simulink model "sl_quadrotor"  (R2024b)
settings: Solver=VariableStepAuto  StartTime=0.0  StopTime=7  RelTol=1e-3  EnableMultiTasking=on
PreLoadFcn:
  | % load parameters of the default quadrotor
  | disp('Quadrotor parameters loaded by PreLoadFcn')
  | mdl_quadrotor
undefined symbols (not defined in the file or in its folder): P, quadrotor, rot2
libraries: simulink x3, roblocks x1, robotcorelib x1, uavutilslib x1
settings Model: Creator=corkep  LastModifiedBy=dawid
settings SolverCC: AlgebraicLoopSolver=TrustRegion
settings DataIOCC: LimitDataPoints=on  ReturnWorkspaceOutputs=off
settings OptimizationCC: ExpressionDepthLimit=2147483647  LifeSpan=inf
settings DebuggingCC: UnderspecifiedInitializationDetection=Classic  MergeDetectMultiDrivingBlocksExec=none  SolverPrmCheckMsg=warning  UnconnectedInputMsg=warning  UnconnectedOutputMsg=warning  UnconnectedLineMsg=warning  AllowSymbolicDim=off  StateNameClashWarn=warning  SFUnexpectedBacktrackingDiag=warning  SFNoUnconditionalDefaultTransitionDiag=warning  SFExecutionAtInitializationDiag=none  ArithmeticOperatorsInVariantConditions=warning
settings HardwareCC: ProdBitPerPointer=32  ProdBitPerSizeT=32  ProdBitPerPtrDiffT=32  ProdLargestAtomicFloat=None  ProdIntDivRoundTo=Undefined  ProdEndianess=Unspecified  ProdWordSize=32  ProdHWDeviceType=32-bit Generic
settings ModelReferenceCC: EnableRefExpFcnMdlSchedulingChecks=on  PropagateSignalLabelsOutOfModel=off
settings SFSimCC: SimUseLocalCustomCode=off  CustomCodeUndefinedFunction=UseInterfaceOnly
settings RTWCC: RTWUseLocalCustomCode=off  GPUComputeCapability=3.5
settings CodeAppCC: StateflowObjectComments=on
settings GRTTargetCC: TargetLangStandard=C89/C90 (ANSI)  CombineOutputUpdateFcns=off  GRTInterface=on
settings ConfigComp: CovMetricSettings=dw  CovSaveCumulativeToWorkspaceVar=on  CovSaveSingleToWorkspaceVar=on  CovExternalEMLEnable=off  CovSFcnEnable=off

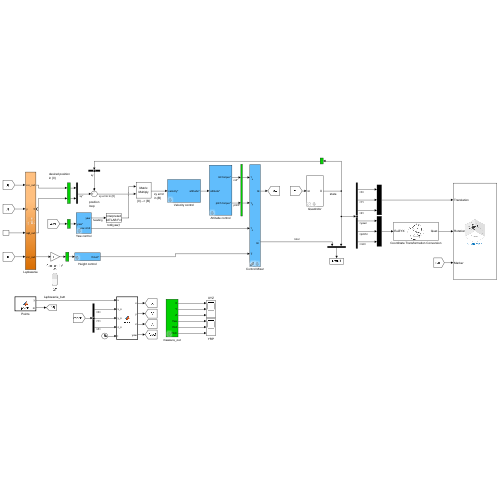
[thumbnail: Simulink's stored preview of the top-level diagram]
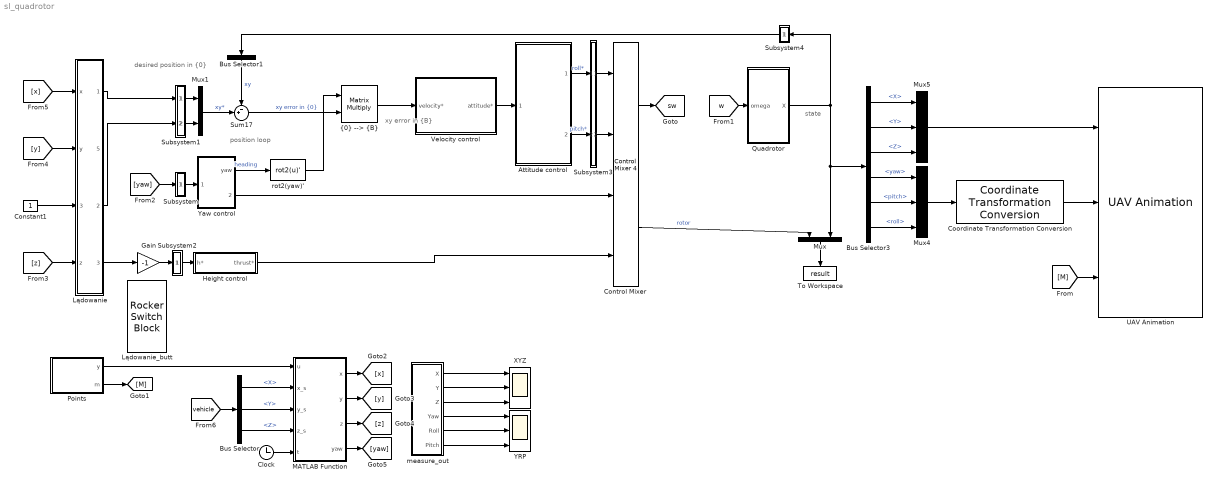
== system sl_quadrotor ==
  note: xy error
      | in {B}
  note: desired position
      | in {0}
  note: position
      | loop
  note: state
  Attitude control : Subsystem  mask{P=50, D=0.08}
      mask prompts: P "Proportional gain"; D "Derivative gain"
  Bus Selector : BusSelector  OutputSignals=X,Y,Z
  Bus Selector1 : BusSelector  OutputSignals=X,Y  OutputAsBus=on
  Bus Selector3 : BusSelector  OutputSignals=X,Y,Z,yaw,pitch,roll
  Clock : Clock
  Constant1 : Constant
  Control Mixer : roblocks/Vehicles/Control Mixer 4  quad=quadrotor  maxrot=5000  minrot=5
  Coordinate Transformation Conversion : robotcorelib/Coordinate Transformation Conversion  InputRepresentation=Euler Angles  InputEulerSequence=ZYX  ShowTrVecInputPort=on  OutputRepresentation=Quaternion  OutputEulerSequence=ZYX  ShowTrVecOutputPort=on  SimulateUsing=Interpreted execution
      settings: LibrarySourceBlock=uavutilslib/Coordinate Transformation Conversion
  Gain : Gain  Gain=-1
  Height control : Subsystem  mask{P=5000, D=0.35, T0=0}
      mask prompts: P "Proportional gain"; D "Derivative gain"; T0 "Thrust feedforward"
  Lądowanie : Subsystem
      settings: PortSchema="{\"entries\":[{\"content\":{\"sides\":[{\"content\":{\"connectorIds\":[\"In1\",\"In2\",\"In3\",\"In4\"]},\"type\":\"ConnectorPlacement.EquallySpacedRectSide\",\"uuid\":\"e16c097e-7f0b-4346-8755-8e731fbb767f\"},{\"content\":{\"connectorIds\":[\"Out1\",\"In5\",\"Out2\",\"Out3\"],\"side\":\"RIGHT\"},\"type\":\"ConnectorPlacement.EquallySpacedRectSide\",\"uuid\":\"595c4242-91f1-4228-8820-ca2fa351ca35\"},{\"content\":{\"side\":\"TOP\"},\"type\":\"ConnectorPlacement.EquallySpacedRectSide\",\"uuid\":\"71163cad-59f2-4c2d-b7f5-2c36c6e60a82\"}]},\"type\":\"ConnectorPlacement.EquallySpacedConnector\",\"uuid\":\"613101b4-3872-4d23-be67-e39dba683d26\"}],\"packageUris\":[\"http://schema.mathworks.com/mf0/Connector/R2020b\"],\"version\":\"1.0\"}"
  Lądowanie_butt : RockerSwitchBlock
      settings: Values={{'Off', 'On'}, [0 1]}
  MATLAB Function : MATLAB Function  TreatAsAtomicUnit=on
  Mux : Mux  Inputs=2
  Mux1 : Mux  Inputs=2
  Mux4 : Mux  Inputs=3
  Mux5 : Mux  Inputs=3
  Points : MATLAB Function  TreatAsAtomicUnit=on
  Quadrotor : Subsystem  AncestorBlock=roblocks/Vehicles/Quadrotor  mask{quad=quadrotor, x0=[0 0 -0.5], groundflag=on}
      mask prompts: quad "Quadrotor params"; x0 "Initial position"; groundflag "Ground"
      mask help: Quadrotor dynamics
      mask Help:
      | Integrate spatial velocity to update pose represented as a homogeneous
      | transformation.
      | 
      | <b>Parameters::</b>
      | 
      | q (struct)  A structure containing quadrotor dynamics
      | 
      | The elements of q are:
      | 
      |  J         Flyer rotational inertia matrix (3x3)
      |  h         Height of rotors above CoG (1x1)
      |  d         Length of flyer arms (1x1)
      |  nb        Number of blades per rotor (1x1)
      |  r         Rotor radius (1x1)
      |  c         Blade chord (1x1)
      |  e         Flapping hinge offset (1x1)
      |  Mb        Rotor blade mass (1x1)
      |  Mc        Estimated hub clamp mass (1x1)
      |  ec        Blade root clamp displacement (1x1)
      |  Ib        Rotor blade rotational inertia (1x1)
      |  Ic        Estimated root clamp inertia (1x1)
      |  mb        Static blade moment (1x1)
      |  Ir        Total rotor inertia (1x1)
      |  Ct        Non-dim. thrust coefficient (1x1)
      |  Cq        Non-dim. torque coefficient (1x1)
      |  sigma     Rotor solidity ratio (1x1)
      |  thetat    Blade tip angle (1x1)
      |  theta0    Blade root angle (1x1)
      |  theta1    Blade twist angle (1x1)
      |  theta75   3/4 blade angle (1x1)
      |  thetai    Blade ideal root approximation (1x1)
      |  a         Lift slope gradient (1x1)
      |  A         Rotor disc area (1x1)
      |  gamma     Lock number (1x1)
      | 
      | 
      | <b>Inputs::</b>
      | 
      | w1 (1x1) angular velocity of rotor 1 [rad]
      | w2 (1x1) angular velocity of rotor 2 [rad]
      | w3 (1x1) angular velocity of rotor 3 [rad]
      | w4 (1x1) angular velocity of rotor 4 [rad]
      | 
      | <b>Outputs::</b>
      | 
      | X (1x12) state vector (x, y, z, thr, thp, thy, xd, yd, zd, thrd, thpd, thyd)
      | 
      | (x,y,z) is the position in the world frame [m]
      | (thr, thp, thy) the roll/pitch/yaw orientation in the world frame [rad]
      | (xd,yd,zd) is the velocity in the body frame [m]
      | (thrd,thpd,thyd) is the roll/pitch/yaw rates in the body frame [rad/s]
      | 
      | <b>Notes::</b>
      | 
      | - See also mdl_quadrotor which defines parameters for the ANU X4 flyer.
      mask Display:
      | port_label('input',1,'\varpi','texmode','on');
      | port_label('output',1,'X','texmode','on');
  Subsystem : Subsystem
      mask DialogControl DescTextVar Prompt: Pomiar zadanego yaw
  Subsystem1 : Subsystem
      mask DialogControl DescTextVar Prompt: Blok pomiarowy wartości zadanych w osi x i y
  Subsystem2 : Subsystem
      mask DialogControl DescTextVar Prompt: Pomiar zadanego yaw
  Subsystem3 : Subsystem
      mask DialogControl DescTextVar Prompt: pomiar zadanego roll pitch
  Subsystem4 : Subsystem
      mask DialogControl DescTextVar Prompt: pomiar sygnałów mierzonych
  Sum17 : Sum  Inputs=-+|
  To Workspace : ToWorkspace  VariableName=result  SampleTime=-1
  UAV Animation : uavutilslib/UAV Animation  NumUAV=1  DynamicUAVConfig=off  UAVType=Multirotor  UAVSize=1  UAVColor=[1 0 0]  UAVTrajectoryAlpha=1  InertialZDirection=Down  RotationFormat=Quaternion  DrawMarkers=on  SampleTime=-1
  Velocity control : Subsystem  mask{P=0.1, D=2}
      mask prompts: P "Proportional gain"; D "Derivative gain"
  XYZ : Scope  NumInputPorts=3
  YRP : Scope  NumInputPorts=3
  Yaw control : Subsystem  mask{P=200, D=1}
      mask prompts: P "Proportional gain"; D "Derivative gain"
  measure_out : Subsystem
      mask DialogControl DescTextVar Prompt: Wyjścia systemu pomiarowego
  rot2(yaw)' : MATLABFcn  MATLABFcn=rot2(u)'  OutputDimensions=[2 2]  Output1D=off
  "{0} --> {B}" : Product  Multiplication=Matrix(*)  RndMeth=Zero
  tag scope: sw=global
  wires:
  Mux/1 -> To Workspace/1
  Control Mixer/2 -> Mux/1  "rotor"
  Sum17/1 -> "{0} --> {B}"/2  "xy error in {0}"
  "{0} --> {B}"/1 -> Velocity control/1(velocity*)
  Mux1/1 -> Sum17/2  "xy*"
  Bus Selector1/1 -> Sum17/1  "xy"
  rot2(yaw)'/1 -> "{0} --> {B}"/1
  Height control/1(thrust*) -> Control Mixer/4
  Bus Selector3/4 -> Mux4/1  "<yaw>"
  Bus Selector3/5 -> Mux4/2  "<pitch>"
  Bus Selector3/6 -> Mux4/3  "<roll>"
  Bus Selector3/3 -> Mux5/3  "<Z>"
  Bus Selector3/2 -> Mux5/2  "<Y>"
  Bus Selector3/1 -> Mux5/1  "<X>"
  Mux4/1 -> Coordinate Transformation Conversion/1
  Coordinate Transformation Conversion/1 -> UAV Animation/2
  Mux5/1 -> UAV Animation/1
  Quadrotor/1(X) -> Subsystem4/1(In1), Bus Selector3/1, Mux/2
  Subsystem1/1(sx_o) -> Mux1/1
  Subsystem1/2(sy_o) -> Mux1/2
  Yaw control/1(yaw) -> rot2(yaw)'/1  "heading"
  Yaw control/2(yaw cmd) -> Control Mixer/3
  Subsystem/1(Out1) -> Yaw control/1(yaw*)
  Subsystem2/1(Out1) -> Height control/1(h*)
  Subsystem4/1(Out1) -> Bus Selector1/1
  measure_out/1(X) -> XYZ/1
  measure_out/2(Y) -> XYZ/2
  measure_out/3(Z) -> XYZ/3
  measure_out/4(Yaw) -> YRP/1
  measure_out/5(Roll) -> YRP/2
  measure_out/6(Pitch) -> YRP/3
  Velocity control/1(attitude*) -> Attitude control/1(attitude*)
  Subsystem3/1(Out1) -> Control Mixer/1
  Attitude control/1(roll torque*) -> Subsystem3/1(In1)  "roll*"
  Subsystem3/2(Out2) -> Control Mixer/2
  Attitude control/2(pitch torque*) -> Subsystem3/2(In2)  "pitch*"
  Gain/1 -> Subsystem2/1(In1)
  [yaw] -> Subsystem/1(In1)
  Control Mixer/1 -> [sw]
  [w] -> Quadrotor/1(omega)
  Constant1/1 -> Lądowanie/3(set)
  Lądowanie/1(x_out) -> Subsystem1/1(sx_in)
  Lądowanie/2(y_out) -> Subsystem1/2(sy_in)
  Lądowanie/3(z_out) -> Gain/1
  Points/2(m) -> [M]
  [M] -> UAV Animation/3
  Points/1(y) -> MATLAB Function/1(u)
  [vehicle] -> Bus Selector/1
  Bus Selector/1 -> MATLAB Function/2(x_s)  "<X>"
  Bus Selector/2 -> MATLAB Function/3(y_s)  "<Y>"
  Bus Selector/3 -> MATLAB Function/4(z_s)  "<Z>"
  Clock/1 -> MATLAB Function/5(t)
  MATLAB Function/1(x) -> [x]
  MATLAB Function/2(y) -> [y]
  MATLAB Function/3(z) -> [z]
  MATLAB Function/4(yaw) -> [yaw]
  [z] -> Lądowanie/4(z)
  [y] -> Lądowanie/2(y)
  [x] -> Lądowanie/1(x)

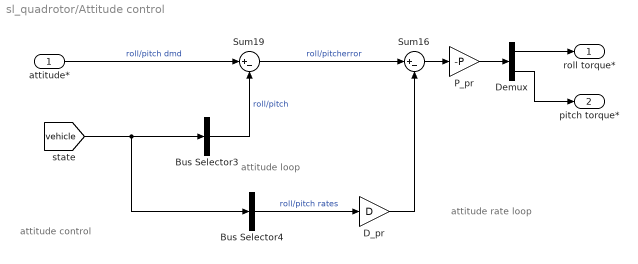
== system sl_quadrotor/Attitude control ==
  note: attitude control
  note: attitude rate loop
  note: attitude loop
  attitude* : Inport
  Bus Selector3 : BusSelector  OutputSignals=roll,pitch  OutputAsBus=on
  Bus Selector4 : BusSelector  OutputSignals=droll,dpitch  OutputAsBus=on
  D_pr : Gain  Gain=D
  Demux : Demux  Outputs=2
  P_pr : Gain  Gain=-P
  Sum16 : Sum  Inputs=|+-
  Sum19 : Sum  Inputs=|+-
  roll torque* : Outport
  pitch torque* : Outport  Port=2
  wires:
  [vehicle] -> Bus Selector4/1, Bus Selector3/1
  attitude*/1 -> Sum19/1  "roll/pitch dmd"
  Bus Selector3/1 -> Sum19/2  "roll/pitch"
  Bus Selector4/1 -> D_pr/1  "roll/pitch rates"
  Sum19/1 -> Sum16/1  "roll/pitcherror"
  Sum16/1 -> P_pr/1
  P_pr/1 -> Demux/1
  D_pr/1 -> Sum16/2
  Demux/2 -> pitch torque*/1
  Demux/1 -> roll torque*/1

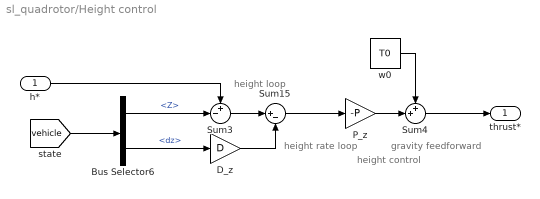
== system sl_quadrotor/Height control ==
  note: height control
  note: gravity feedforward
  note: height rate
      | loop
  note: height
      | loop
  h* : Inport
  Bus Selector6 : BusSelector  OutputSignals=Z,dz
  D_z : Gain  Gain=D
  P_z : Gain  Gain=-P
  Sum15 : Sum  Inputs=|+-
  Sum3 : Sum  Inputs=+-|
  Sum4 : Sum  Inputs=++|
  w0 : Constant  Value=T0  SampleTime=0
  thrust* : Outport
  wires:
  w0/1 -> Sum4/1
  Sum15/1 -> P_z/1
  P_z/1 -> Sum4/2
  Bus Selector6/1 -> Sum3/2  "<Z>"
  h*/1 -> Sum3/1
  Sum3/1 -> Sum15/1
  Bus Selector6/2 -> D_z/1  "<dz>"
  D_z/1 -> Sum15/2
  Sum4/1 -> thrust*/1
  [vehicle] -> Bus Selector6/1

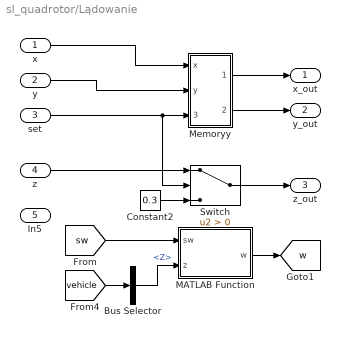
== system sl_quadrotor/Lądowanie ==
  x : Inport
  y : Inport  Port=2
  set : Inport  Port=3
  z : Inport  Port=4
  In5 : Inport  Port=5
  Bus Selector : BusSelector  OutputSignals=Z
  Constant2 : Constant  Value=0.3
  MATLAB Function : MATLAB Function  TreatAsAtomicUnit=on
  Memoryy : Subsystem
  Switch : Switch  Criteria=u2 > Threshold  SaturateOnIntegerOverflow=off  InputSameDT=off
  x_out : Outport
  y_out : Outport  Port=2
  z_out : Outport  Port=3
  tag scope: w=global
  wires:
  Bus Selector/1 -> MATLAB Function/2(z)  "<Z>"
  [vehicle] -> Bus Selector/1
  Constant2/1 -> Switch/3
  set/1 -> Memoryy/3(set), Switch/2
  Memoryy/2(Out2) -> y_out/1
  [sw] -> MATLAB Function/1(sw)
  Memoryy/1(Out1) -> x_out/1
  MATLAB Function/1(w) -> [w]
  y/1 -> Memoryy/2(y)
  z/1 -> Switch/1
  x/1 -> Memoryy/1(x)
  Switch/1 -> z_out/1

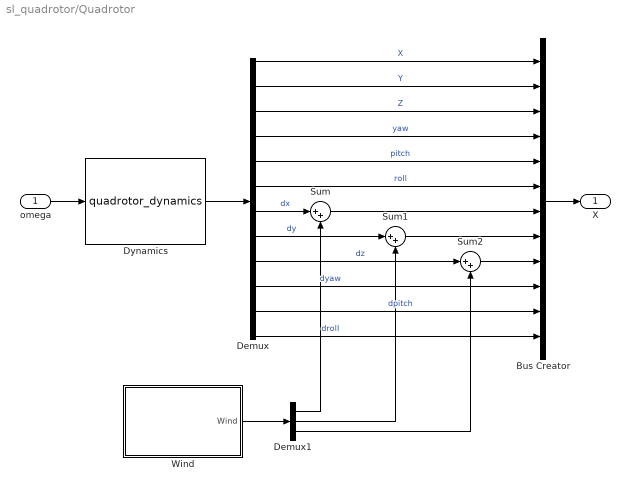
== system sl_quadrotor/Quadrotor ==
  omega : Inport
  Bus Creator : BusCreator  Inputs='X','Y','Z','yaw','pitch','roll','dx','dy','dz','dyaw','dpitch','droll'
  Demux : Demux  Outputs=12
      settings: DisplayOption=none
  Demux1 : Demux  Outputs=3
  Dynamics : S-Function  FunctionName=quadrotor_dynamics  Parameters=quad, x0, groundflag  SFunctionDeploymentMode=off  EnableBusSupport=off
  Sum : Sum  Inputs=|++
  Sum1 : Sum  Inputs=|++
  Sum2 : Sum  Inputs=|++
  Wind : Subsystem
  X : Outport
  wires:
  Demux/1 -> Bus Creator/1  "X"
  Demux/3 -> Bus Creator/3  "Z"
  Demux/4 -> Bus Creator/4  "yaw"
  Demux/5 -> Bus Creator/5  "pitch"
  omega/1 -> Dynamics/1
  Demux/2 -> Bus Creator/2  "Y"
  Demux/6 -> Bus Creator/6  "roll"
  Bus Creator/1 -> X/1
  Dynamics/1 -> Demux/1
  Demux/10 -> Bus Creator/10  "dyaw"
  Demux/11 -> Bus Creator/11  "dpitch"
  Demux/12 -> Bus Creator/12  "droll"
  Sum2/1 -> Bus Creator/9
  Demux/9 -> Sum2/1  "dz"
  Sum1/1 -> Bus Creator/8
  Demux/8 -> Sum1/1  "dy"
  Demux/7 -> Sum/1  "dx"
  Sum/1 -> Bus Creator/7
  Demux1/1 -> Sum/2
  Demux1/2 -> Sum1/2
  Demux1/3 -> Sum2/2
  Wind/1(Wind) -> Demux1/1

== system sl_quadrotor/Subsystem ==
  In1 : Inport
  Out1 : Outport
  tag scope: syaw=global
  wires:
  In1/1 -> Out1/1, [syaw]

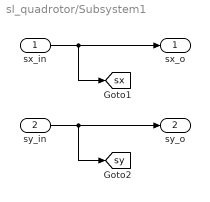
== system sl_quadrotor/Subsystem1 ==
  sx_in : Inport
  sy_in : Inport  Port=2
  sx_o : Outport
  sy_o : Outport  Port=2
  tag scope: sx=global, sy=global
  wires:
  sx_in/1 -> sx_o/1, [sx]
  sy_in/1 -> sy_o/1, [sy]

== system sl_quadrotor/Subsystem2 ==
  In1 : Inport
  Out1 : Outport
  tag scope: sz=global
  wires:
  In1/1 -> [sz], Out1/1

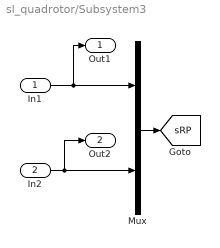
== system sl_quadrotor/Subsystem3 ==
  In1 : Inport
  In2 : Inport  Port=2
  Mux : Mux  Inputs=2
  Out1 : Outport
  Out2 : Outport  Port=2
  tag scope: sRP=global
  wires:
  Mux/1 -> [sRP]
  In1/1 -> Out1/1, Mux/1
  In2/1 -> Out2/1, Mux/2

== system sl_quadrotor/Subsystem4 ==
  In1 : Inport
  Out1 : Outport
  tag scope: vehicle=global
  wires:
  In1/1 -> Out1/1, [vehicle]

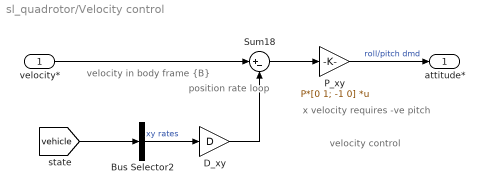
== system sl_quadrotor/Velocity control ==
  note: x velocity requires -ve pitch
  note: velocity in body frame {B}
  note: velocity control
  note: position rate
      | loop
  velocity* : Inport
  Bus Selector2 : BusSelector  OutputSignals=dx,dy  OutputAsBus=on
  D_xy : Gain  Gain=D
  P_xy : Gain  Gain=P*[0 1; -1 0]  Multiplication=Matrix(K*u)
  Sum18 : Sum  Inputs=|+-
  attitude* : Outport
  wires:
  Bus Selector2/1 -> D_xy/1  "xy rates"
  D_xy/1 -> Sum18/2
  Sum18/1 -> P_xy/1
  velocity*/1 -> Sum18/1
  [vehicle] -> Bus Selector2/1
  P_xy/1 -> attitude*/1  "roll/pitch dmd"

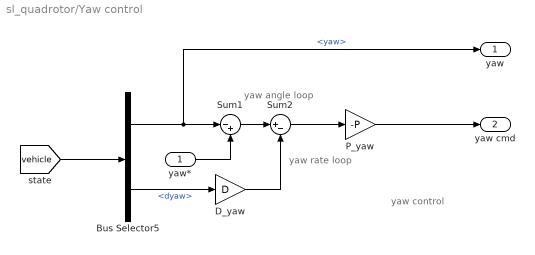
== system sl_quadrotor/Yaw control ==
  note: yaw control
  note: yaw rate
      | loop
  note: yaw angle
      | loop
  yaw* : Inport
  Bus Selector5 : BusSelector  OutputSignals=yaw,dyaw
  D_yaw : Gain  Gain=D
  P_yaw : Gain  Gain=-P
  Sum1 : Sum  Inputs=|-+
  Sum2 : Sum  Inputs=|+-
  yaw : Outport
  yaw cmd : Outport  Port=2
  wires:
  [vehicle] -> Bus Selector5/1
  P_yaw/1 -> yaw cmd/1
  Bus Selector5/1 -> Sum1/1, yaw/1  "<yaw>"
  Sum2/1 -> P_yaw/1
  Bus Selector5/2 -> D_yaw/1  "<dyaw>"
  D_yaw/1 -> Sum2/2
  Sum1/1 -> Sum2/1
  yaw*/1 -> Sum1/2

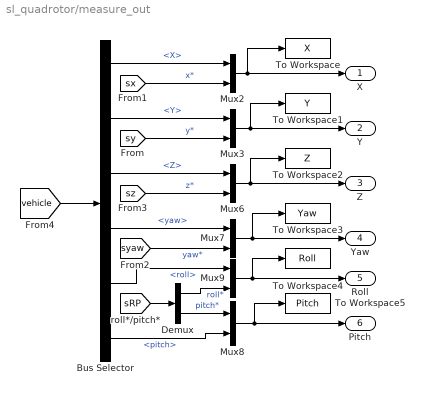
== system sl_quadrotor/measure_out ==
  Bus Selector : BusSelector  OutputSignals=X,Y,Z,yaw,roll,pitch
  Demux : Demux  Outputs=2
  Mux{2..3,6..9} (6 alike) : Mux  Inputs=2
  To Workspace : ToWorkspace  VariableName=X  SaveFormat=Structure With Time  SampleTime=-1
  To Workspace1 : ToWorkspace  VariableName=Y  SaveFormat=Structure With Time  SampleTime=-1
      settings: Save2DSignal=2-D array (concatenate along first dimension)
  To Workspace2 : ToWorkspace  VariableName=Z  SaveFormat=Structure With Time  SampleTime=-1
      settings: Save2DSignal=2-D array (concatenate along first dimension)
  To Workspace3 : ToWorkspace  VariableName=Yaw  SaveFormat=Structure With Time  SampleTime=-1
      settings: Save2DSignal=2-D array (concatenate along first dimension)
  To Workspace4 : ToWorkspace  VariableName=Roll  SaveFormat=Structure With Time  SampleTime=-1
      settings: Save2DSignal=2-D array (concatenate along first dimension)
  To Workspace5 : ToWorkspace  VariableName=Pitch  SaveFormat=Structure With Time  SampleTime=-1
      settings: Save2DSignal=2-D array (concatenate along first dimension)
  X : Outport
  Y : Outport  Port=2
  Z : Outport  Port=3
  Yaw : Outport  Port=4
  Roll : Outport  Port=5
  Pitch : Outport  Port=6
  wires:
  [sx] -> Mux2/2  "x*"
  Bus Selector/4 -> Mux7/1  "<yaw>"
  Bus Selector/3 -> Mux6/1  "<Z>"
  Mux2/1 -> To Workspace/1, X/1
  [vehicle] -> Bus Selector/1
  Bus Selector/2 -> Mux3/1  "<Y>"
  Demux/2 -> Mux8/1  "pitch*"
  [syaw] -> Mux7/2  "yaw*"
  [sz] -> Mux6/2  "z*"
  Bus Selector/1 -> Mux2/1  "<X>"
  [sy] -> Mux3/2  "y*"
  Demux/1 -> Mux9/2  "roll*"
  Bus Selector/5 -> Mux9/1  "<roll>"
  [sRP] -> Demux/1
  Bus Selector/6 -> Mux8/2  "<pitch>"
  Mux9/1 -> To Workspace4/1, Roll/1
  Mux8/1 -> To Workspace5/1, Pitch/1
  Mux7/1 -> To Workspace3/1, Yaw/1
  Mux6/1 -> To Workspace2/1, Z/1
  Mux3/1 -> To Workspace1/1, Y/1

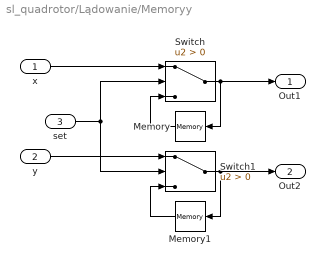
== system sl_quadrotor/Lądowanie/Memoryy ==
  x : Inport
  y : Inport  Port=2
  set : Inport  Port=3
  Memory : Memory
  Memory1 : Memory
  Switch : Switch  Criteria=u2 > Threshold  SaturateOnIntegerOverflow=off  InputSameDT=off
  Switch1 : Switch  Criteria=u2 > Threshold  SaturateOnIntegerOverflow=off  InputSameDT=off
  Out1 : Outport
  Out2 : Outport  Port=2
  wires:
  Switch/1 -> Out1/1, Memory/1
  y/1 -> Switch1/1
  Memory1/1 -> Switch1/3
  Memory/1 -> Switch/3
  Switch1/1 -> Out2/1, Memory1/1
  x/1 -> Switch/1
  set/1 -> Switch1/2, Switch/2

== system sl_quadrotor/Quadrotor/Wind ==
  Constant1 : Constant  Value=[0; 0; 0]
  Constant2 : Constant  Value=[P.wind_n; P.wind_e; P.wind_d]
  Sum : Sum  Inputs=|++
  Wind Gusts : Subsystem
  Wind : Outport
  wires:
  Constant2/1 -> Sum/1
  Wind Gusts/1(gusts) -> Sum/2
  Sum/1 -> Wind/1

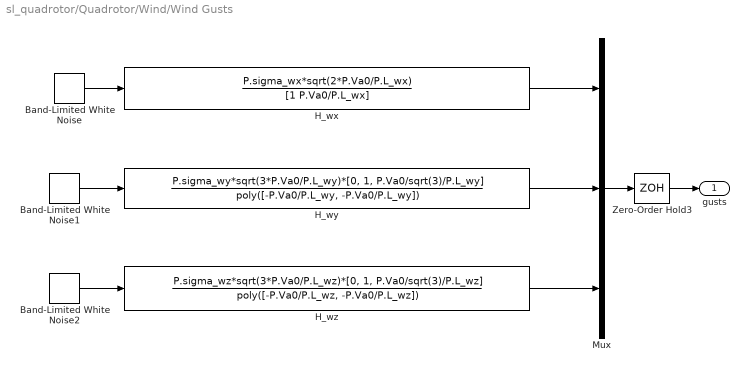
== system sl_quadrotor/Quadrotor/Wind/Wind Gusts ==
  Band-Limited White Noise : simulink/Sources/Band-Limited White Noise  Cov=[1]  Ts=P.Ts  seed=[23341]
  Band-Limited White Noise1 : simulink/Sources/Band-Limited White Noise  Cov=[1]  Ts=P.Ts  seed=[23341]
  Band-Limited White Noise2 : simulink/Sources/Band-Limited White Noise  Cov=[1]  Ts=P.Ts  seed=[23341]
  H_wx : TransferFcn  Numerator=P.sigma_wx*sqrt(2*P.Va0/P.L_wx)  Denominator=[1 P.Va0/P.L_wx]
  H_wy : TransferFcn  Numerator=P.sigma_wy*sqrt(3*P.Va0/P.L_wy)*[0, 1, P.Va0/sqrt(3)/P.L_wy]  Denominator=poly([-P.Va0/P.L_wy, -P.Va0/P.L_wy])
  H_wz : TransferFcn  Numerator=P.sigma_wz*sqrt(3*P.Va0/P.L_wz)*[0, 1, P.Va0/sqrt(3)/P.L_wz]  Denominator=poly([-P.Va0/P.L_wz, -P.Va0/P.L_wz])
  Mux : Mux  Inputs=3
  Zero-Order Hold3 : ZeroOrderHold  SampleTime=-1
  gusts : Outport
  wires:
  H_wx/1 -> Mux/1
  Band-Limited White Noise/1 -> H_wx/1
  H_wy/1 -> Mux/2
  Band-Limited White Noise1/1 -> H_wy/1
  H_wz/1 -> Mux/3
  Band-Limited White Noise2/1 -> H_wz/1
  Mux/1 -> Zero-Order Hold3/1
  Zero-Order Hold3/1 -> gusts/1

== matlab function sl_quadrotor/Points ==
  data: y output; m output
function [y, m] = points()
persistent P T;

if isempty(P)
    % ---- x --- y --- z --- yaw --- time----
    P = [  1,    1,    1,     1,      0.5; ...
           2,    1,    3,     0.5,    0.5; ...
          -1,    2,    2,    -0.5,    0.5];
end

if isempty(T)
    T = [  1,    1,    -1; ...
           2,    1,    -3; ...
           -1,   2,    -2];
end

y = P;
m = T;

== matlab function sl_quadrotor/Lądowanie/MATLAB Function ==
  data: sw input; w output; z input
function w = fcn(sw,z)

    if (z > -0.35) && (z < -0.30)
        w = 0.8*sw;
    elseif (z >= -0.30) && (z < -0.20)
        w = 0.6*sw;
    elseif (z >= -0.20)
        w = 0.1*sw;
    else
        w = sw;
    end

== matlab function sl_quadrotor/MATLAB Function ==
  settings: updateMethod=DISCRETE  sampleTime=0.01
  data: x output; u input; y output; z output; yaw output; x_s input; y_s input; z_s input; t input
function [x, y, z, yaw] = way(u, x_s, y_s, z_s, t)

persistent i
persistent start_time

if isempty(i)
    i = 1;
end

if isempty(start_time)
    start_time = t;
end

       
        x = u(i, 1);
        y = u(i, 2);
        z = u(i, 3);
        yaw = u(i, 4);
        w_time = u(i,5);

        distance = sqrt((x - x_s)^2 + (y - y_s)^2 + (z + z_s)^2);
        disp(sprintf('Distance: %.3f', distance))
        if distance < 0.1
            elapsed_time = t - start_time;
            disp(sprintf('Start time: %.3f', start_time))
            disp(sprintf('Elapsed time: %.3f', elapsed_time))
            if elapsed_time >= w_time
                i = i+1;
                if i >= height(u)
                    i  = height(u);
                end
                disp("waypoint")

            end
        else
            start_time = t;
        end
   
end
